simulink model "Enceinte_climatique"  (R2025b)
settings: Solver=VariableStepAuto  StartTime=0.0  StopTime=6  RelTol=1e-3
settings Model: Creator=boiteth  LastModifiedBy=rofte

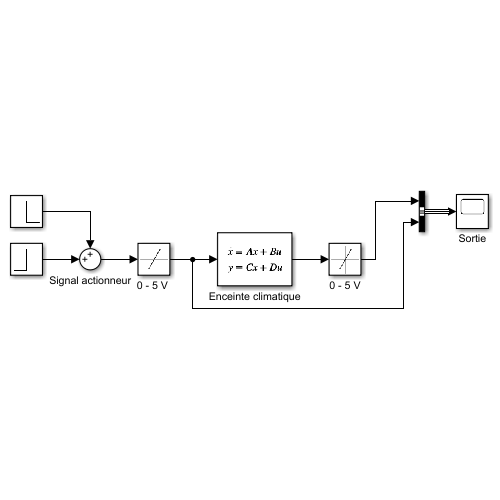
[thumbnail: Simulink's stored preview of the top-level diagram]
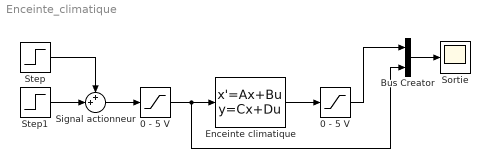
== system Enceinte_climatique ==
  0 - 5 V : Saturate  UpperLimit=5  LowerLimit=0  LinearizeAsGain=off
  "0 - 5 V " : Saturate  UpperLimit=5  LowerLimit=0
  Bus Creator : BusCreator  Inputs=2
  Enceinte climatique : StateSpace  A=-2  B=2  D=0  InitialCondition=0
  Signal actionneur : Sum  Inputs=++|
  Sortie : Scope
      settings: ActiveDisplayYMinimum=-3.644200174510388  ActiveDisplayYMaximum=5.9014912360284031
  Step : Step  Time=4  After=-0.5  SampleTime=0
  Step1 : Step  Time=0.5  Before=1.66  After=2.33  SampleTime=0
  wires:
  Bus Creator/1 -> Sortie/1
  Step1/1 -> Signal actionneur/2
  Step/1 -> Signal actionneur/1
  Signal actionneur/1 -> "0 - 5 V "/1
  "0 - 5 V "/1 -> Bus Creator/2, Enceinte climatique/1
  0 - 5 V/1 -> Bus Creator/1
  Enceinte climatique/1 -> 0 - 5 V/1
